simulink model "Navid_SynchGen7th_Order_model"  (R2017b)
settings: Solver=ode45  StartTime=0.0  StopTime=30  EnableMultiTasking=on
libraries: simulink x2
settings Model: Creator=NAVIDG  LastModifiedBy=NAVIDG
settings DataIOCC: LimitDataPoints=on  SaveFormat=Array  SignalLoggingSaveFormat=ModelDataLogs
settings OptimizationCC: InitFltsAndDblsToZero=on  LifeSpan=inf
settings DebuggingCC: SaveWithParameterizedLinksMsg=none  UnderspecifiedInitializationDetection=Classic  MergeDetectMultiDrivingBlocksExec=none  SignalResolutionControl=TryResolveAllWithWarning  SolverPrmCheckMsg=warning  MultiTaskDSMMsg=warning  MultiTaskCondExecSysMsg=none  SFUnexpectedBacktrackingDiag=warning  SFNoUnconditionalDefaultTransitionDiag=warning  SFExecutionAtInitializationDiag=none
settings HardwareCC: ProdBitPerPointer=32  ProdBitPerSizeT=32  ProdBitPerPtrDiffT=32  ProdLargestAtomicFloat=None  ProdIntDivRoundTo=Undefined  ProdEndianess=Unspecified  ProdWordSize=32  ProdHWDeviceType=32-bit Generic
settings ModelReferenceCC: PropagateSignalLabelsOutOfModel=off
settings CodeAppCC: StateflowObjectComments=on
settings GRTTargetCC: TargetFcnLib=ansi_tfl_tmw.mat  TargetLangStandard=C89/C90 (ANSI)  CombineOutputUpdateFcns=off  GRTInterface=on
settings ConfigComp: CovMetricSettings=dw  CovHtmlReporting=on  CovSaveCumulativeToWorkspaceVar=on  CovSaveSingleToWorkspaceVar=on  CovExternalEMLEnable=off

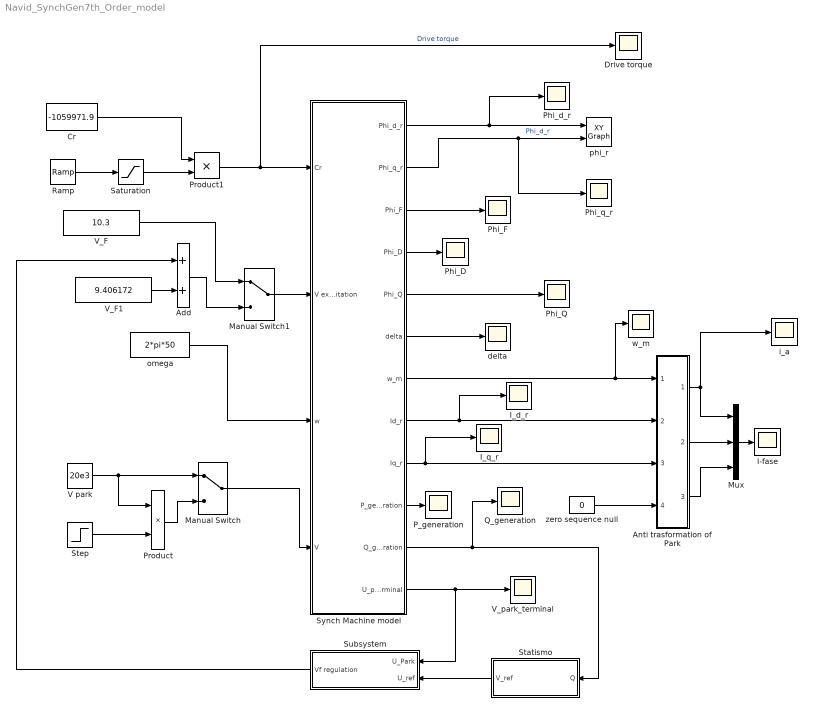
== system Navid_SynchGen7th_Order_model ==
  Add : Sum
  Anti trasformation of Park : Subsystem
  Cr : Constant  Value=-1059971.9
  Drive torque : Scope
  I-fase : Scope
  I_d_r : Scope
  I_q_r : Scope
  Manual Switch : ManualSwitch
  Manual Switch1 : ManualSwitch
  Mux : Mux  Inputs=3
  P_generation : Scope
  Phi_D : Scope
  Phi_F : Scope
  Phi_Q : Scope
  Phi_d_r : Scope
  Phi_q_r : Scope
  Product : Product  RndMeth=Zero
  Product1 : Product  RndMeth=Zero
  Q_generation : Scope
  Ramp : simulink/Sources/Ramp  slope=0.05  start=15  X0=0
  Saturation : Saturate  UpperLimit=0.25
  Statismo : Subsystem
  Step : Step  Before=1  After=0  SampleTime=1
  Subsystem : Subsystem
  Synch Machine model : Subsystem  mask{Ld=7e-3, Ll=0.35*2.25/(2*pi*50), Lm=6.6659e-3, L_D=8.7419e-3, L_F=7.3835e-3, Lq=5.61e-3, Mq=4.7704e-3, Rs=1.6e-3, RF=9.845e-4, RD=0.11558, RQ=0.0204, n=1, J=2.812e4}
      mask prompts: Ll "L linea"; L_D "LD"; L_F "LF"; n "Num coppie polari"; J "Inerzia"
  V park : Constant  Value=20e3
  V_F : Constant  Value=10.3
  V_F1 : Constant  Value=9.406172
  V_park_terminal : Scope
  delta : Scope
  i_a : Scope
  omega : Constant  Value=2*pi*50
  phi_r : simulink/Sinks/XY Graph  xmin=-60  xmax=60  ymin=-60  ymax=60  st=-1
  w_m : Scope
  zero sequence null : Constant  Value=0
  wires:
  omega/1 -> Synch Machine model/3(w)
  Manual Switch/1 -> Synch Machine model/4(V)
  V park/1 -> Manual Switch/1, Product/1
  Step/1 -> Product/2
  Product/1 -> Manual Switch/2
  Synch Machine model/8(Id_r) -> Anti trasformation of Park/2(i_d), I_d_r/1
  Synch Machine model/1(Phi_d_r) -> phi_r/1, Phi_d_r/1  "Phi_d_r"
  Synch Machine model/2(Phi_q_r) -> phi_r/2, Phi_q_r/1
  Synch Machine model/3(Phi_F) -> Phi_F/1
  Synch Machine model/4(Phi_D) -> Phi_D/1
  Synch Machine model/5(Phi_Q) -> Phi_Q/1
  Synch Machine model/6(delta) -> delta/1
  Synch Machine model/7(w_m) -> w_m/1, Anti trasformation of Park/1(wp)
  Synch Machine model/9(Iq_r) -> Anti trasformation of Park/3(i_q), I_q_r/1
  zero sequence null/1 -> Anti trasformation of Park/4(i_o)
  Anti trasformation of Park/1(i_a) -> Mux/1, i_a/1
  Anti trasformation of Park/2(i_b) -> Mux/2
  Anti trasformation of Park/3(i_c) -> Mux/3
  Mux/1 -> I-fase/1
  Ramp/1 -> Saturation/1
  Saturation/1 -> Product1/2
  Cr/1 -> Product1/1
  Product1/1 -> Drive torque/1, Synch Machine model/1(Cr)  "Drive torque"
  Synch Machine model/12(U_park_terminal) -> Subsystem/1(U_Park), V_park_terminal/1
  Subsystem/1(Vf regulation) -> Add/1
  Manual Switch1/1 -> Synch Machine model/2(V excitation)
  V_F/1 -> Manual Switch1/1
  Add/1 -> Manual Switch1/2
  V_F1/1 -> Add/2
  Statismo/1(V_ref) -> Subsystem/2(U_ref)
  Synch Machine model/11(Q_generation) -> Statismo/1(Q), Q_generation/1
  Synch Machine model/10(P_generation) -> P_generation/1

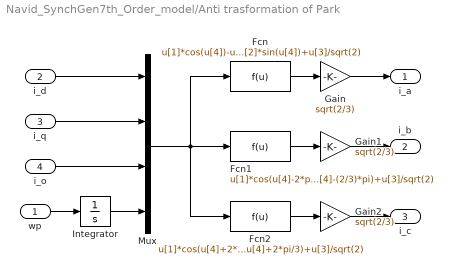
== system Navid_SynchGen7th_Order_model/Anti trasformation of Park ==
  wp : Inport
  i_d : Inport  Port=2
  i_q : Inport  Port=3
  i_o : Inport  Port=4
  Fcn : Fcn  Expr=u[1]*cos(u[4])-u[2]*sin(u[4])+u[3]/sqrt(2)
  Fcn1 : Fcn  Expr=u[1]*cos(u[4]-2*pi/3)-u[2]*sin(u[4]-(2/3)*pi)+u[3]/sqrt(2)
  Fcn2 : Fcn  Expr=u[1]*cos(u[4]+2*pi/3)-u[2]*sin(u[4]+2*pi/3)+u[3]/sqrt(2)
  Gain : Gain  Gain=sqrt(2/3)  SaturateOnIntegerOverflow=on  OutDataTypeStr=Inherit: Same as input  ParamDataTypeStr=Inherit: Same as input
  Gain1 : Gain  Gain=sqrt(2/3)  SaturateOnIntegerOverflow=on  OutDataTypeStr=Inherit: Same as input  ParamDataTypeStr=Inherit: Same as input
  Gain2 : Gain  Gain=sqrt(2/3)  SaturateOnIntegerOverflow=on  OutDataTypeStr=Inherit: Same as input  ParamDataTypeStr=Inherit: Same as input
  Integrator : Integrator
  Mux : Mux
  i_a : Outport
  i_b : Outport  Port=2
  i_c : Outport  Port=3
  wires:
  i_d/1 -> Mux/1
  i_q/1 -> Mux/2
  i_o/1 -> Mux/3
  Mux/1 -> Fcn/1, Fcn1/1, Fcn2/1
  wp/1 -> Integrator/1
  Integrator/1 -> Mux/4
  Fcn2/1 -> Gain2/1
  Fcn1/1 -> Gain1/1
  Fcn/1 -> Gain/1
  Gain/1 -> i_a/1
  Gain1/1 -> i_b/1
  Gain2/1 -> i_c/1

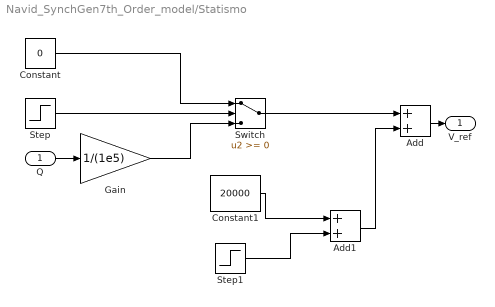
== system Navid_SynchGen7th_Order_model/Statismo ==
  Q : Inport
  Add : Sum
  Add1 : Sum
  Constant : Constant  Value=0
  Constant1 : Constant  Value=20000
  Gain : Gain  Gain=1/(1e5)
  Step : Step  Time=75  After=-1  SampleTime=0
  Step1 : Step  Time=0  After=500  SampleTime=0
  Switch : Switch
  V_ref : Outport
  wires:
  Q/1 -> Gain/1
  Step/1 -> Switch/2
  Gain/1 -> Switch/3
  Constant/1 -> Switch/1
  Switch/1 -> Add/1
  Constant1/1 -> Add1/1
  Step1/1 -> Add1/2
  Add1/1 -> Add/2
  Add/1 -> V_ref/1

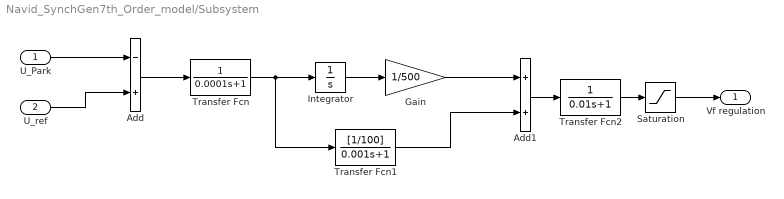
== system Navid_SynchGen7th_Order_model/Subsystem ==
  U_Park : Inport
  U_ref : Inport  Port=2
  Add : Sum  Inputs=-+
  Add1 : Sum
  Gain : Gain  Gain=1/500
  Integrator : Integrator
  Saturation : Saturate  UpperLimit=15  LowerLimit=-10
  Transfer Fcn : TransferFcn  Denominator=[0.0001 1]
  Transfer Fcn1 : TransferFcn  Numerator=[1/100]  Denominator=[0.001 1]
  Transfer Fcn2 : TransferFcn  Denominator=[0.01 1]
  Vf regulation : Outport
  wires:
  U_Park/1 -> Add/1
  U_ref/1 -> Add/2
  Add/1 -> Transfer Fcn/1
  Transfer Fcn/1 -> Integrator/1, Transfer Fcn1/1
  Integrator/1 -> Gain/1
  Gain/1 -> Add1/1
  Transfer Fcn1/1 -> Add1/2
  Add1/1 -> Transfer Fcn2/1
  Transfer Fcn2/1 -> Saturation/1
  Saturation/1 -> Vf regulation/1

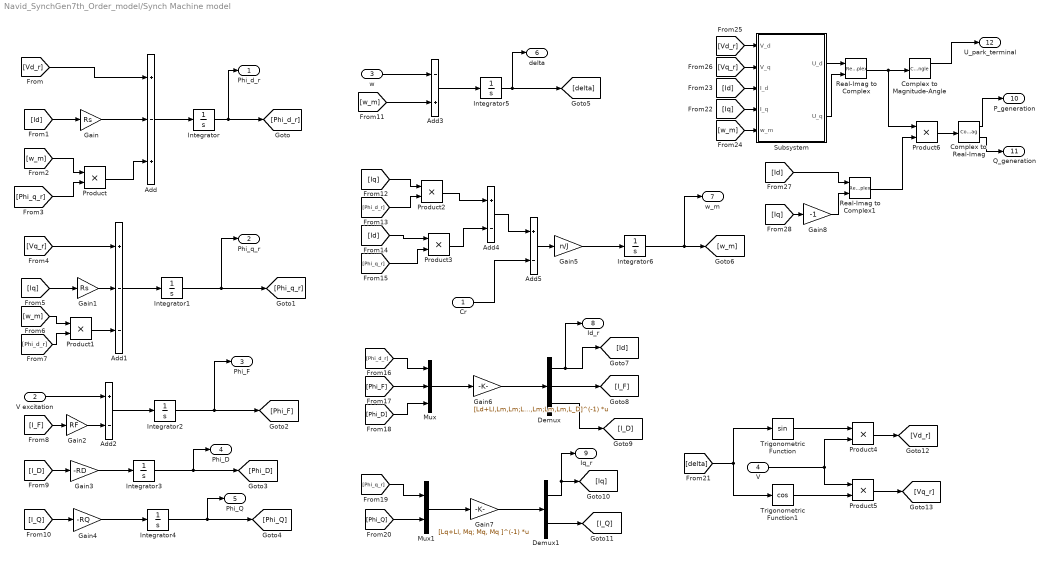
== system Navid_SynchGen7th_Order_model/Synch Machine model ==
  Cr : Inport
  V excitation : Inport  Port=2
  w : Inport  Port=3
  V : Inport  Port=4
  Add : Sum  Inputs=+-+
  Add1 : Sum  Inputs=+--
  Add2 : Sum  Inputs=+-
  Add3 : Sum  Inputs=-+
  Add4 : Sum  Inputs=+-
  Add5 : Sum  Inputs=+-
  Complex to Magnitude-Angle : ComplexToMagnitudeAngle
  Complex to Real-Imag : ComplexToRealImag
  Demux : Demux  Outputs=3
  Demux1 : Demux  Outputs=2
  Gain : Gain  Gain=Rs
  Gain1 : Gain  Gain=Rs
  Gain2 : Gain  Gain=RF
  Gain3 : Gain  Gain=-RD
  Gain4 : Gain  Gain=-RQ
  Gain5 : Gain  Gain=n/J
  Gain6 : Gain  Gain=[Ld+Ll,Lm,Lm;Lm,L_F,Lm;Lm,Lm,L_D]^(-1)  Multiplication=Matrix(K*u)
  Gain7 : Gain  Gain=[Lq+Ll, Mq; Mq, Mq ]^(-1)  Multiplication=Matrix(K*u)
  Gain8 : Gain  Gain=-1
  Integrator : Integrator  InitialCondition=63.662
  Integrator1 : Integrator
  Integrator2 : Integrator  InitialCondition=70.621
  Integrator3 : Integrator  InitialCondition=63.662
  Integrator4 : Integrator
  Integrator5 : Integrator
  Integrator6 : Integrator  InitialCondition=2*pi*50
  Mux : Mux  Inputs=3
  Mux1 : Mux  Inputs=2
  Product{,1..6} (7 alike) : Product  RndMeth=Zero
  Real-Imag to Complex : RealImagToComplex
  Real-Imag to Complex1 : RealImagToComplex
  Subsystem : Subsystem  mask{Ll=0.35*2.25/(2*pi*50)}
  Trigonometric Function : Trigonometry
  Trigonometric Function1 : Trigonometry  Operator=cos
  Phi_d_r : Outport
  Phi_q_r : Outport  Port=2
  Phi_F : Outport  Port=3
  Phi_D : Outport  Port=4
  Phi_Q : Outport  Port=5
  delta : Outport  Port=6
  w_m : Outport  Port=7
  Id_r : Outport  Port=8
  Iq_r : Outport  Port=9
  P_generation : Outport  Port=10
  Q_generation : Outport  Port=11
  U_park_terminal : Outport  Port=12
  wires:
  [w_m] -> Product/1
  [Phi_q_r] -> Product/2
  [Id] -> Gain/1
  Product/1 -> Add/3
  Gain/1 -> Add/2
  [Vd_r] -> Add/1
  Add/1 -> Integrator/1
  Integrator/1 -> [Phi_d_r], Phi_d_r/1
  [Vq_r] -> Add1/1
  Gain1/1 -> Add1/2
  [Iq] -> Gain1/1
  [w_m] -> Product1/1
  [Phi_d_r] -> Product1/2
  Product1/1 -> Add1/3
  Add1/1 -> Integrator1/1
  Integrator1/1 -> [Phi_q_r], Phi_q_r/1
  V excitation/1 -> Add2/1
  [I_F] -> Gain2/1
  Gain2/1 -> Add2/2
  Add2/1 -> Integrator2/1
  Integrator2/1 -> [Phi_F], Phi_F/1
  [I_D] -> Gain3/1
  Gain3/1 -> Integrator3/1
  Integrator3/1 -> [Phi_D], Phi_D/1
  Gain4/1 -> Integrator4/1
  Integrator4/1 -> [Phi_Q], Phi_Q/1
  [I_Q] -> Gain4/1
  w/1 -> Add3/1
  [w_m] -> Add3/2
  Add3/1 -> Integrator5/1
  Integrator5/1 -> [delta], delta/1
  [Iq] -> Product2/1
  [Phi_d_r] -> Product2/2
  [Id] -> Product3/1
  [Phi_q_r] -> Product3/2
  Product2/1 -> Add4/1
  Product3/1 -> Add4/2
  Add4/1 -> Add5/1
  Cr/1 -> Add5/2
  Add5/1 -> Gain5/1
  Gain5/1 -> Integrator6/1
  Integrator6/1 -> [w_m], w_m/1
  [Phi_d_r] -> Mux/1
  [Phi_F] -> Mux/2
  [Phi_D] -> Mux/3
  Mux/1 -> Gain6/1
  Gain6/1 -> Demux/1
  Demux/1 -> [Id], Id_r/1
  Demux/2 -> [I_F]
  Demux/3 -> [I_D]
  [Phi_q_r] -> Mux1/1
  [Phi_Q] -> Mux1/2
  Mux1/1 -> Gain7/1
  Gain7/1 -> Demux1/1
  Demux1/1 -> [Iq], Iq_r/1
  Demux1/2 -> [I_Q]
  [delta] -> Trigonometric Function/1, Trigonometric Function1/1
  V/1 -> Product4/2, Product5/1
  Trigonometric Function/1 -> Product4/1
  Trigonometric Function1/1 -> Product5/2
  Product4/1 -> [Vd_r]
  Product5/1 -> [Vq_r]
  [Iq] -> Subsystem/4(I_q)
  [Id] -> Subsystem/3(I_d)
  [w_m] -> Subsystem/5(w_m)
  [Vd_r] -> Subsystem/1(V_d)
  [Vq_r] -> Subsystem/2(V_q)
  Subsystem/1(U_d) -> Real-Imag to Complex/1
  Subsystem/2(U_q) -> Real-Imag to Complex/2
  Real-Imag to Complex/1 -> Complex to Magnitude-Angle/1, Product6/1
  [Id] -> Real-Imag to Complex1/1
  [Iq] -> Gain8/1
  Gain8/1 -> Real-Imag to Complex1/2
  Real-Imag to Complex1/1 -> Product6/2
  Product6/1 -> Complex to Real-Imag/1
  Complex to Real-Imag/1 -> P_generation/1
  Complex to Real-Imag/2 -> Q_generation/1
  Complex to Magnitude-Angle/1 -> U_park_terminal/1

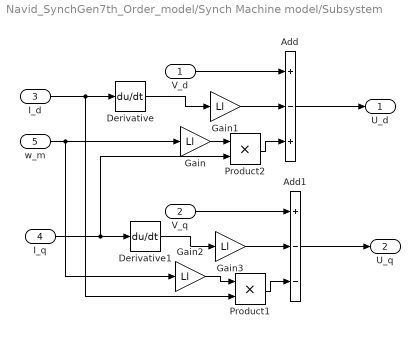
== system Navid_SynchGen7th_Order_model/Synch Machine model/Subsystem ==
  V_d : Inport
  V_q : Inport  Port=2
  I_d : Inport  Port=3
  I_q : Inport  Port=4
  w_m : Inport  Port=5
  Add : Sum  Inputs=+-+
  Add1 : Sum  Inputs=+--
  Derivative : Derivative
  Derivative1 : Derivative
  Gain{,1..3} (4 alike) : Gain  Gain=Ll
  Product1 : Product  RndMeth=Zero
  Product2 : Product  RndMeth=Zero
  U_d : Outport
  U_q : Outport  Port=2
  wires:
  V_d/1 -> Add/1
  w_m/1 -> Gain/1, Gain2/1
  I_d/1 -> Derivative/1, Product1/2
  Derivative/1 -> Gain1/1
  Gain1/1 -> Add/2
  Add/1 -> U_d/1
  V_q/1 -> Add1/1
  I_q/1 -> Derivative1/1, Product2/2
  Derivative1/1 -> Gain3/1
  Gain3/1 -> Add1/2
  Add1/1 -> U_q/1
  Gain/1 -> Product2/1
  Product2/1 -> Add/3
  Gain2/1 -> Product1/1
  Product1/1 -> Add1/3
